simulink model "Task4"  (R2025b)
settings: Solver=ode4  StartTime=0.0  StopTime=100  FixedStep=1/100  RelTol=1e-6
undefined symbols (not defined in the file): mode
settings Model: Creator=antony  LastModifiedBy=Antony

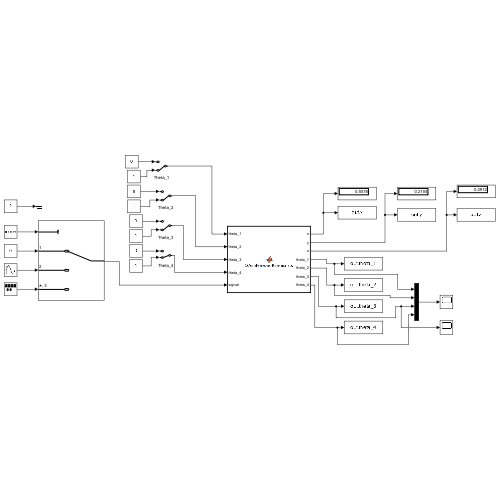
[thumbnail: Simulink's stored preview of the top-level diagram]
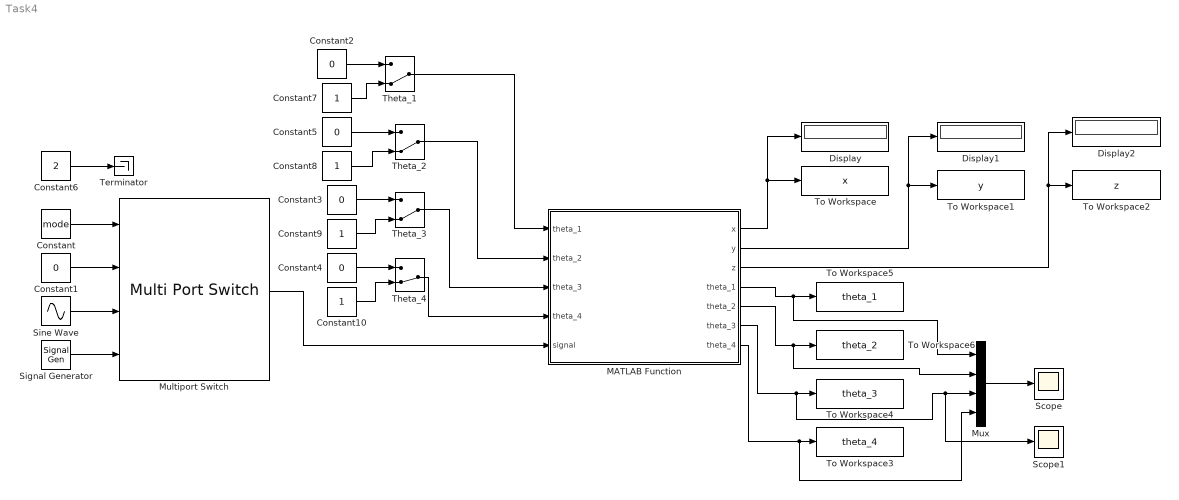
== system Task4 ==
  Constant : Constant  Value=mode
  Constant{1..5} (5 alike) : Constant  Value=0
  Constant{7..10} (4 alike) : Constant
  Constant6 : Constant  Value=2
  Display : Display
  Display1 : Display
  Display2 : Display
  MATLAB Function : MATLAB Function  TreatAsAtomicUnit=on
  Multiport Switch : MultiPortSwitch  SaturateOnIntegerOverflow=off  InputSameDT=off
  Mux : Mux
  Scope : Scope
      settings: ActiveDisplayYMinimum=-1  ActiveDisplayYMaximum=1
  Scope1 : Scope
      settings: ActiveDisplayYMinimum=-0.49087385212340517  ActiveDisplayYMaximum=0.49087385212340517
  Signal Generator : SignalGenerator  WaveForm=square  Amplitude=pi/8  Units=rad/sec
  Sine Wave : Sin  Amplitude=pi/8  Frequency=pi/4  SampleTime=0
  Terminator : Terminator
  Theta_{1..4} (4 alike) : ManualSwitch  CurrentSetting=0
  To Workspace : ToWorkspace  VariableName=x  SampleTime=-1
  To Workspace1 : ToWorkspace  VariableName=y  SampleTime=-1
  To Workspace2 : ToWorkspace  VariableName=z  SampleTime=-1
  To Workspace3 : ToWorkspace  VariableName=theta_4  SampleTime=-1
  To Workspace4 : ToWorkspace  VariableName=theta_3  SampleTime=-1
  To Workspace5 : ToWorkspace  VariableName=theta_1  SampleTime=-1
  To Workspace6 : ToWorkspace  VariableName=theta_2  SampleTime=-1
  wires:
  Sine Wave/1 -> Multiport Switch/3
  Constant1/1 -> Multiport Switch/2
  Signal Generator/1 -> Multiport Switch/4
  Constant2/1 -> Theta_1/1
  Constant3/1 -> Theta_3/1
  Constant4/1 -> Theta_4/1
  Constant5/1 -> Theta_2/1
  MATLAB Function/1(x) -> To Workspace/1, Display/1
  MATLAB Function/2(y) -> Display1/1, To Workspace1/1
  MATLAB Function/3(z) -> Display2/1, To Workspace2/1
  MATLAB Function/4(theta_1) -> Mux/1, To Workspace5/1
  MATLAB Function/5(theta_2) -> Mux/2, To Workspace6/1
  MATLAB Function/6(theta_3) -> Scope1/1, Mux/3, To Workspace4/1
  MATLAB Function/7(theta_4) -> To Workspace3/1, Mux/4
  Mux/1 -> Scope/1
  Constant6/1 -> Terminator/1
  Constant/1 -> Multiport Switch/1
  Constant7/1 -> Theta_1/2
  Constant8/1 -> Theta_2/2
  Constant9/1 -> Theta_3/2
  Constant10/1 -> Theta_4/2
  Multiport Switch/1 -> MATLAB Function/5(signal)
  Theta_4/1 -> MATLAB Function/4("theta_4 ")
  Theta_3/1 -> MATLAB Function/3("theta_3 ")
  Theta_2/1 -> MATLAB Function/2("theta_2 ")
  Theta_1/1 -> MATLAB Function/1("theta_1 ")

== matlab function Task4/MATLAB Function ==
  data: x output; theta_1 input; y output; theta_2 input; theta_3 input; theta_4 input; z output; theta_1 output; theta_2 output; theta_3 output; theta_4 output; signal input
function [x,y,z,theta_1, theta_2, theta_3,theta_4]= QArmForwardKinematics(theta_1, theta_2, theta_3,theta_4, signal)

    theta_1 = theta_1*signal;
    if theta_2 ~= 0
        theta_3 = 0;
    else
        theta_3 = theta_3*signal;
    end
    theta_2 = theta_2*signal;
    theta_4 = theta_4*signal;


    L1 = 0.14;
    L2 = 0.35;
    L3 = 0.05;
    L4 = 0.25;
    L5 = 0.15;

    T04 = [sin(theta_1)*sin(theta_4) + cos(theta_1)*cos(theta_2)*cos(theta_4)*sin(theta_3) + cos(theta_1)*cos(theta_3)*cos(theta_4)*sin(theta_2), ...
        cos(theta_4)*sin(theta_1) - cos(theta_1)*cos(theta_2)*sin(theta_3)*sin(theta_4) - cos(theta_1)*cos(theta_3)*sin(theta_2)*sin(theta_4), ...
        cos(theta_2 + theta_3)*cos(theta_1), cos(theta_1)*sin(theta_2 + atan(L3/L2))*sqrt(L2^2 + L3^2) + cos(theta_2 + theta_3)*cos(theta_1)*(L4 + L5); ...
        cos(theta_2)*cos(theta_4)*sin(theta_1)*sin(theta_3) - cos(theta_1)*sin(theta_4) + cos(theta_3)*cos(theta_4)*sin(theta_1)*sin(theta_2), ...
        - cos(theta_1)*cos(theta_4) - cos(theta_2)*sin(theta_1)*sin(theta_3)*sin(theta_4) - cos(theta_3)*sin(theta_1)*sin(theta_2)*sin(theta_4), ...
        cos(theta_2 + theta_3)*sin(theta_1), sin(theta_1)*sin(theta_2 + atan(L3/L2))*sqrt(L2^2 + L3^2) + cos(theta_2 + theta_3)*sin(theta_1)*(L4 + L5); ...
        cos(theta_2 + theta_3)*cos(theta_4), -cos(theta_2 + theta_3)*sin(theta_4), -sin(theta_2 + theta_3), ...
        -(L2^2*L4*sin(theta_2 + theta_3) - L1*L3^2 - L1*L2^2 + L2^2*L5*sin(theta_2 + theta_3) + L3^2*L4*sin(theta_2 + theta_3) + L3^2*L5*sin(theta_2 + theta_3) ...
        - L2^2*cos(theta_2)*sqrt(L2^2 + L3^2)*sqrt((L2^2 + L3^2)/L2^2) + L2*L3*sin(theta_2)*sqrt(L2^2 + L3^2)*sqrt((L2^2 + L3^2)/L2^2))/(L2^2 + L3^2); 0, 0, 0, 1];
    x = T04(1,4);
    y = T04(2,4);
    z = T04(3,4);


end
